simulink model "ex9busSG_sim"  (R2014b)
settings: Solver=ode45  SolverMode=SingleTasking  StartTime=0.0  StopTime=6  MaxStep=0.006  RelTol=1e-05
values from neighbouring files (symbols this model uses):
  Ar = full(Ar)    [ex9busSG.m]
  baseA = baseVA/baseV    [ex14busSGandPV.m]    (also in ex9busSG.m; exDroopA.m = baseVA./baseV; exDroopB.m = baseVA./baseV; exLargeSysStability.m = baseVA./baseV)
  baseV = 1e3*mpcA.bus(1,BASE_KV)    [ex14busSGandPV.m]    (also in ex9busSG_data.mat = 345000; exDroopA.m = 1e3*mpc.bus(:,BASE_KV); exDroopB.m = 1e3*mpc.bus(:,BASE_KV); exLargeSysStability.m = 1e3*mpc.bus(:,BASE_KV))
  baseVA = mpcA.baseMVA * 1e6    [ex14busSGandPV.m]    (also in ex9busSG.m = mpc.baseMVA*1e6; exDroopA.m = mpc.baseMVA * 1e6; exDroopB.m = mpc.baseMVA * 1e6; exLargeSysStability.m = mpc.baseMVA * 1e6)
  Br = full(Br)    [ex9busSG.m]
  Cr = full(Cr)    [ex9busSG.m]
  delta_init = mpc.bus(Genbus,VA)*pi/180    [ex9busSG.m]
  Dr = full(Dr)    [ex9busSG.m]
  Genbus = Genbus(2:end)    [ex9busSG.m]
  Kd = KD_GAIN_CNST*J*ws    [ex14busSGandPV.m]    (also in ex2busStability.m = 24000; ex7busLongLine.m; ex9busSG.m; exDroopA.m)
  lamda = (2^0.5) * Vgmag/ws    (= 45.916132124)    [ex2busStability.m]    (also in ex9busSG.m = (2^0.5) * Vn_gens/ws)
  MM = length(ssbus)    [ex9busSG.m]    (also in exLargeSysStability.m)
  poles_2Jws = poles./(2*J*ws)    [ex14busSGandPV.m]    (also in ex2busStability.m = poles./(2*ws*J); ex7busLongLine.m; ex9busSG.m = poles./(2*ws*J); exDroopA.m)
  ppm_default = (3*Pn_gens)    [ex9busSG.m]
  ppm_step_size_W = ppm_rel_step*Pmax_gens(which_generator_to_step)    [ex9busSG.m]
  ppm_step_time = 2    [ex9busSG.m]
  ref_vd_MKS = (2^0.5)*real(VV1ph)    [ex9busSG.m]
  ref_vq_MKS = (2^0.5)*imag(VV1ph)    [ex9busSG.m]
  ws = 2*pi*50    (= 314.159265359)    [ex14busSGandPV.m]    (also in ex2busStability.m; ex3busPV.m; ex7busLongLine.m; ex9busSG.m)
libraries: simulink x2
settings Model: Creator=COPEC  LastModifiedBy=Juri
settings OptimizationCC: BlockReduction=off  BooleanDataType=off
settings DebuggingCC: SaveWithParameterizedLinksMsg=none  UnderspecifiedInitializationDetection=Classic  MergeDetectMultiDrivingBlocksExec=none  SignalResolutionControl=TryResolveAllWithWarning  SolverPrmCheckMsg=none  FrameProcessingCompatibilityMsg=error
settings HardwareCC: TargetUnknown=on

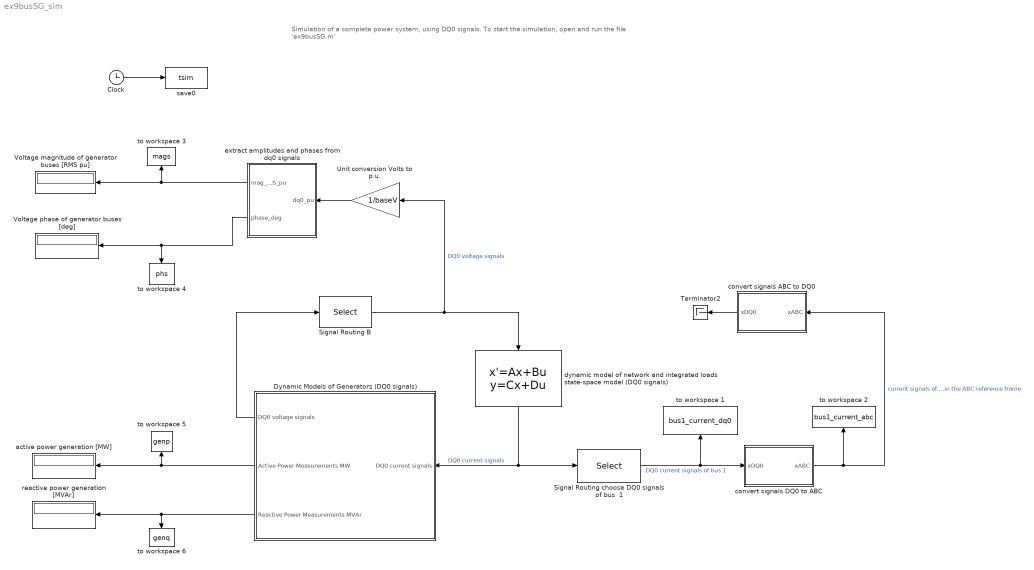
== system ex9busSG_sim ==
  note: Simulation of a complete power system, using DQ0 signals.
      |
      | To start the simulation, open and run the file
      | 'ex9busSG.m'
  Clock : Clock
  Dynamic Models of Generators (DQ0 signals) : Subsystem
  "Signal Routing choose DQ0 signals of bus  1 " : Selector  InputPortWidth=3*MM  IndexOptions=Index vector (dialog)  Indices=Bus_to_Ref  OutputSizes=1
  Signal Routing B : Selector  InputPortWidth=3*MM  IndexOptions=Index vector (dialog)  Indices=Units_to_Net  OutputSizes=1
  Terminator2 : Terminator
  Unit conversion Volts to p.u. : Gain  Gain=1/baseV
  Voltage magnitude of generator buses [RMS pu] : Display
  Voltage phase of generator buses [deg] : Display
  active power generation [MW] : Display
  convert signals ABC to DQ0 : Subsystem
  convert signals DQ0 to ABC : Subsystem
  dynamic model of network and integrated loads state-space model (DQ0 signals) : StateSpace  A=Ar  B=Br  C=Cr  D=Dr  X0=0
  extract amplitudes and phases from dq0 signals : Subsystem
  reactive power generation [MVAr] : Display
  save0 : ToWorkspace  VariableName=tsim  SampleTime=-1
  to workspace 1 : ToWorkspace  VariableName=bus1_current_dq0  SampleTime=-1
  to workspace 2 : ToWorkspace  VariableName=bus1_current_abc  SampleTime=-1
  to workspace 3 : ToWorkspace  VariableName=mags  SampleTime=-1
  to workspace 4 : ToWorkspace  VariableName=phs  SampleTime=-1
  to workspace 5 : ToWorkspace  VariableName=genp  SampleTime=-1
  to workspace 6 : ToWorkspace  VariableName=genq  SampleTime=-1
  wires:
  Clock/1 -> save0/1
  extract amplitudes and phases from dq0 signals/2(phase_deg) -> to workspace 4/1, Voltage phase of generator buses [deg]/1
  extract amplitudes and phases from dq0 signals/1(mag_RMS_pu) -> to workspace 3/1, Voltage magnitude of generator buses [RMS pu]/1
  Unit conversion Volts to p.u./1 -> extract amplitudes and phases from dq0 signals/1(dq0_pu)
  dynamic model of network and integrated loads state-space model (DQ0 signals)/1 -> "Signal Routing choose DQ0 signals of bus  1 "/1, Dynamic Models of Generators (DQ0 signals)/1(DQ0 current signals)  "DQ0 current signals"
  Signal Routing B/1 -> Unit conversion Volts to p.u./1, dynamic model of network and integrated loads state-space model (DQ0 signals)/1  "DQ0 voltage signals"
  "Signal Routing choose DQ0 signals of bus  1 "/1 -> convert signals DQ0 to ABC/1(xDQ0), to workspace 1/1  "DQ0 current signals of bus 1"
  convert signals DQ0 to ABC/1(xABC) -> convert signals ABC to DQ0/1(xABC), to workspace 2/1  "current signals of bus 1 in the ABC reference frame"
  convert signals ABC to DQ0/1(xDQ0) -> Terminator2/1
  Dynamic Models of Generators (DQ0 signals)/3(Reactive Power Measurements MVAr) -> reactive power generation [MVAr]/1, to workspace 6/1
  Dynamic Models of Generators (DQ0 signals)/2(Active Power Measurements MW) -> active power generation [MW]/1, to workspace 5/1
  Dynamic Models of Generators (DQ0 signals)/1(DQ0 voltage signals) -> Signal Routing B/1

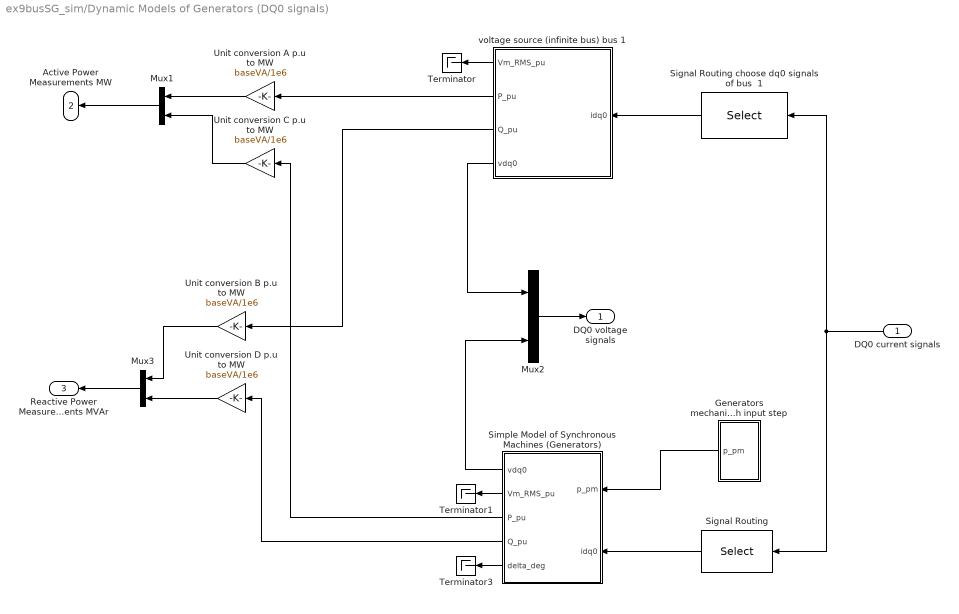
== system ex9busSG_sim/Dynamic Models of Generators (DQ0 signals) ==
  DQ0 current signals : Inport
  Generators mechanical powers with input step : Subsystem
  Mux1 : Mux  Inputs=2
  Mux2 : Mux  Inputs=2
  Mux3 : Mux  Inputs=2
  Signal Routing : Selector  InputPortWidth=3*MM  IndexOptions=Index vector (dialog)  Indices=Bus_to_Gen  OutputSizes=1
  "Signal Routing choose dq0 signals of bus  1 " : Selector  InputPortWidth=3*MM  IndexOptions=Index vector (dialog)  Indices=Bus_to_Ref  OutputSizes=1
  Simple Model of Synchronous Machines (Generators) : Subsystem
  Terminator : Terminator
  Terminator1 : Terminator
  Terminator3 : Terminator
  Unit conversion A p.u to MW : Gain  Gain=baseVA/1e6
  Unit conversion B p.u to MW : Gain  Gain=baseVA/1e6
  Unit conversion C p.u to MW : Gain  Gain=baseVA/1e6
  Unit conversion D p.u to MW : Gain  Gain=baseVA/1e6
  voltage source (infinite bus) bus 1 : Subsystem
  DQ0 voltage signals : Outport
  Active Power Measurements MW : Outport  Port=2
  Reactive Power Measurements MVAr : Outport  Port=3
  wires:
  voltage source (infinite bus) bus 1/2(P_pu) -> Unit conversion A p.u to MW/1
  Simple Model of Synchronous Machines (Generators)/4(Q_pu) -> Unit conversion D p.u to MW/1
  voltage source (infinite bus) bus 1/1(Vm_RMS_pu) -> Terminator/1
  Mux2/1 -> DQ0 voltage signals/1
  Signal Routing/1 -> Simple Model of Synchronous Machines (Generators)/2(idq0)
  voltage source (infinite bus) bus 1/4(vdq0) -> Mux2/1
  Simple Model of Synchronous Machines (Generators)/1(vdq0) -> Mux2/2
  "Signal Routing choose dq0 signals of bus  1 "/1 -> voltage source (infinite bus) bus 1/1(idq0)
  Unit conversion A p.u to MW/1 -> Mux1/1
  Unit conversion B p.u to MW/1 -> Mux3/1
  Simple Model of Synchronous Machines (Generators)/5(delta_deg) -> Terminator3/1
  Simple Model of Synchronous Machines (Generators)/2(Vm_RMS_pu) -> Terminator1/1
  Mux3/1 -> Reactive Power Measurements MVAr/1
  Unit conversion D p.u to MW/1 -> Mux3/2
  Unit conversion C p.u to MW/1 -> Mux1/2
  Mux1/1 -> Active Power Measurements MW/1
  Simple Model of Synchronous Machines (Generators)/3(P_pu) -> Unit conversion C p.u to MW/1
  DQ0 current signals/1 -> "Signal Routing choose dq0 signals of bus  1 "/1, Signal Routing/1
  voltage source (infinite bus) bus 1/3(Q_pu) -> Unit conversion B p.u to MW/1
  Generators mechanical powers with input step/1(p_pm) -> Simple Model of Synchronous Machines (Generators)/1(p_pm)

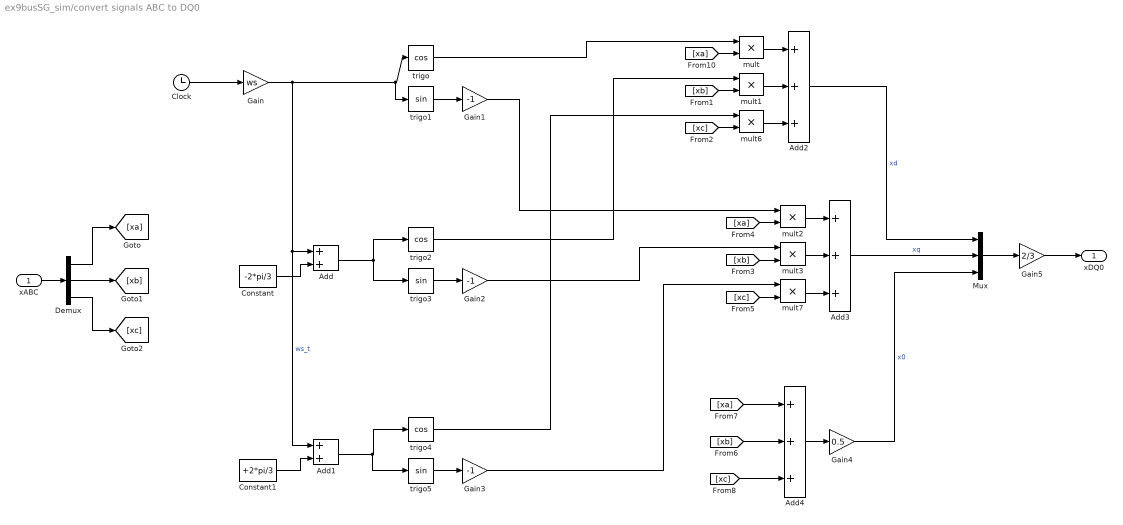
== system ex9busSG_sim/convert signals ABC to DQ0 ==
  xABC : Inport
  Add : Sum
  Add1 : Sum
  Add2 : Sum  Inputs=+++
  Add3 : Sum  Inputs=+++
  Add4 : Sum  Inputs=+++
  Clock : Clock
  Constant : Constant  Value=-2*pi/3
  Constant1 : Constant  Value=+2*pi/3
  Demux : Demux  Outputs=3
  Gain : Gain  Gain=ws
  Gain1 : Gain  Gain=-1
  Gain2 : Gain  Gain=-1
  Gain3 : Gain  Gain=-1
  Gain4 : Gain  Gain=0.5
  Gain5 : Gain  Gain=2/3
  Mux : Mux  Inputs=3
  mult{,1..3,6..7} (6 alike) : Product  Inputs=**
  trigo : Trigonometry  Operator=cos
  trigo1 : Trigonometry
  trigo2 : Trigonometry  Operator=cos
  trigo3 : Trigonometry
  trigo4 : Trigonometry  Operator=cos
  trigo5 : Trigonometry
  xDQ0 : Outport
  wires:
  Clock/1 -> Gain/1
  Gain/1 -> trigo1/1, trigo/1, Add1/1, Add/1  "ws_t"
  Constant/1 -> Add/2
  Constant1/1 -> Add1/2
  trigo1/1 -> Gain1/1
  trigo3/1 -> Gain2/1
  Add/1 -> trigo2/1, trigo3/1
  trigo5/1 -> Gain3/1
  Add1/1 -> trigo5/1, trigo4/1
  xABC/1 -> Demux/1
  Demux/1 -> [xa]
  Demux/2 -> [xb]
  Demux/3 -> [xc]
  mult/1 -> Add2/1
  mult1/1 -> Add2/2
  [xa] -> mult/2
  [xb] -> mult1/2
  mult2/1 -> Add3/1
  mult3/1 -> Add3/2
  Add2/1 -> Mux/1  "xd"
  Add3/1 -> Mux/2  "xq"
  Gain4/1 -> Mux/3  "x0"
  trigo/1 -> mult/1
  trigo2/1 -> mult1/1
  [xc] -> mult6/2
  mult6/1 -> Add2/3
  trigo4/1 -> mult6/1
  [xa] -> mult2/2
  [xb] -> mult3/2
  [xc] -> mult7/2
  mult7/1 -> Add3/3
  Add4/1 -> Gain4/1
  [xa] -> Add4/1
  [xb] -> Add4/2
  [xc] -> Add4/3
  Gain1/1 -> mult2/1
  Gain2/1 -> mult3/1
  Gain3/1 -> mult7/1
  Mux/1 -> Gain5/1
  Gain5/1 -> xDQ0/1

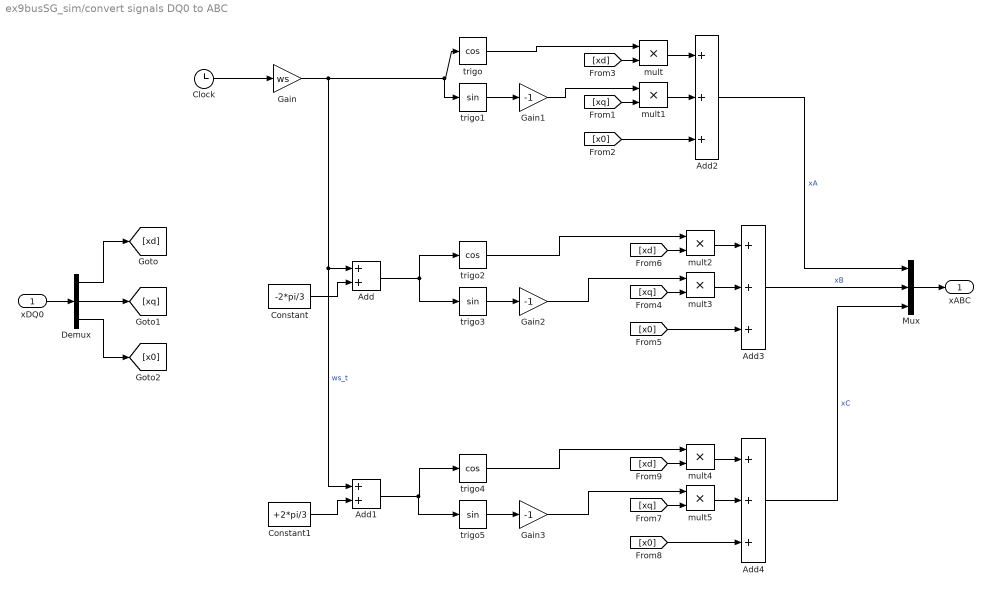
== system ex9busSG_sim/convert signals DQ0 to ABC ==
  xDQ0 : Inport
  Add : Sum
  Add1 : Sum
  Add2 : Sum  Inputs=+++
  Add3 : Sum  Inputs=+++
  Add4 : Sum  Inputs=+++
  Clock : Clock
  Constant : Constant  Value=-2*pi/3
  Constant1 : Constant  Value=+2*pi/3
  Demux : Demux  Outputs=3
  Gain : Gain  Gain=ws
  Gain1 : Gain  Gain=-1
  Gain2 : Gain  Gain=-1
  Gain3 : Gain  Gain=-1
  Mux : Mux  Inputs=3
  mult{,1..5} (6 alike) : Product  Inputs=**
  trigo : Trigonometry  Operator=cos
  trigo1 : Trigonometry
  trigo2 : Trigonometry  Operator=cos
  trigo3 : Trigonometry
  trigo4 : Trigonometry  Operator=cos
  trigo5 : Trigonometry
  xABC : Outport
  wires:
  Clock/1 -> Gain/1
  Gain/1 -> trigo1/1, trigo/1, Add1/1, Add/1  "ws_t"
  Constant/1 -> Add/2
  Constant1/1 -> Add1/2
  trigo1/1 -> Gain1/1
  trigo3/1 -> Gain2/1
  Add/1 -> trigo2/1, trigo3/1
  trigo5/1 -> Gain3/1
  Add1/1 -> trigo5/1, trigo4/1
  xDQ0/1 -> Demux/1
  Demux/1 -> [xd]
  Demux/2 -> [xq]
  Demux/3 -> [x0]
  Mux/1 -> xABC/1
  mult/1 -> Add2/1
  mult1/1 -> Add2/2
  [xd] -> mult/2
  [xq] -> mult1/2
  [x0] -> Add2/3
  mult2/1 -> Add3/1
  mult3/1 -> Add3/2
  [xd] -> mult2/2
  [xq] -> mult3/2
  [x0] -> Add3/3
  mult4/1 -> Add4/1
  mult5/1 -> Add4/2
  [xd] -> mult4/2
  [xq] -> mult5/2
  [x0] -> Add4/3
  trigo/1 -> mult/1
  Gain1/1 -> mult1/1
  trigo2/1 -> mult2/1
  Gain2/1 -> mult3/1
  trigo4/1 -> mult4/1
  Gain3/1 -> mult5/1
  Add2/1 -> Mux/1  "xA"
  Add3/1 -> Mux/2  "xB"
  Add4/1 -> Mux/3  "xC"

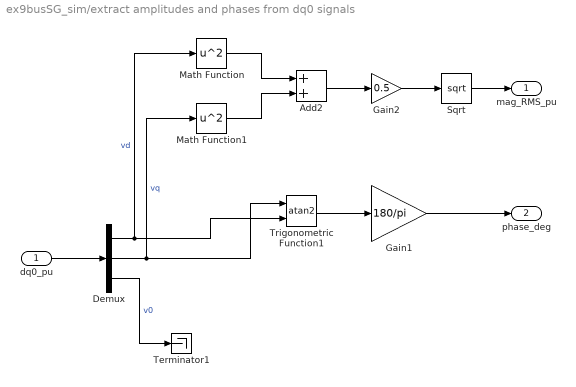
== system ex9busSG_sim/extract amplitudes and phases from dq0 signals ==
  dq0_pu : Inport
  Add2 : Sum
  Demux : Demux  Outputs=3
  Gain1 : Gain  Gain=180/pi
  Gain2 : Gain  Gain=0.5
  Math Function : Math  Operator=square  SaturateOnIntegerOverflow=on
  Math Function1 : Math  Operator=square  SaturateOnIntegerOverflow=on
  Sqrt : Sqrt  SaturateOnIntegerOverflow=on
  Terminator1 : Terminator
  Trigonometric Function1 : Trigonometry  Operator=atan2
  mag_RMS_pu : Outport
  phase_deg : Outport  Port=2
  wires:
  dq0_pu/1 -> Demux/1
  Demux/1 -> Trigonometric Function1/2, Math Function/1  "vd"
  Demux/2 -> Trigonometric Function1/1, Math Function1/1  "vq"
  Demux/3 -> Terminator1/1  "v0"
  Sqrt/1 -> mag_RMS_pu/1
  Math Function/1 -> Add2/1
  Math Function1/1 -> Add2/2
  Add2/1 -> Gain2/1
  Gain2/1 -> Sqrt/1
  Trigonometric Function1/1 -> Gain1/1
  Gain1/1 -> phase_deg/1

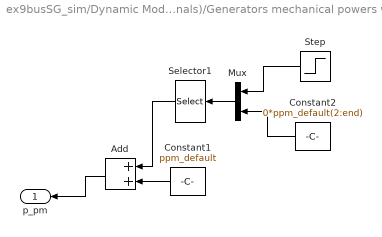
== system ex9busSG_sim/Dynamic Models of Generators (DQ0 signals)/Generators mechanical powers with input step ==
  Add : Sum
  Constant1 : Constant  Value=ppm_default
  Constant2 : Constant  Value=0*ppm_default(2:end)
  Mux : Mux  Inputs=2
  Selector1 : Selector  InputPortWidth=length(ppm_default)  IndexOptions=Index vector (dialog)  Indices=step_index_vector  OutputSizes=1
  Step : Step  Time=ppm_step_time  After=ppm_step_size_W  SampleTime=0
  p_pm : Outport
  wires:
  Constant1/1 -> Add/2
  Selector1/1 -> Add/1
  Constant2/1 -> Mux/2
  Mux/1 -> Selector1/1
  Step/1 -> Mux/1
  Add/1 -> p_pm/1

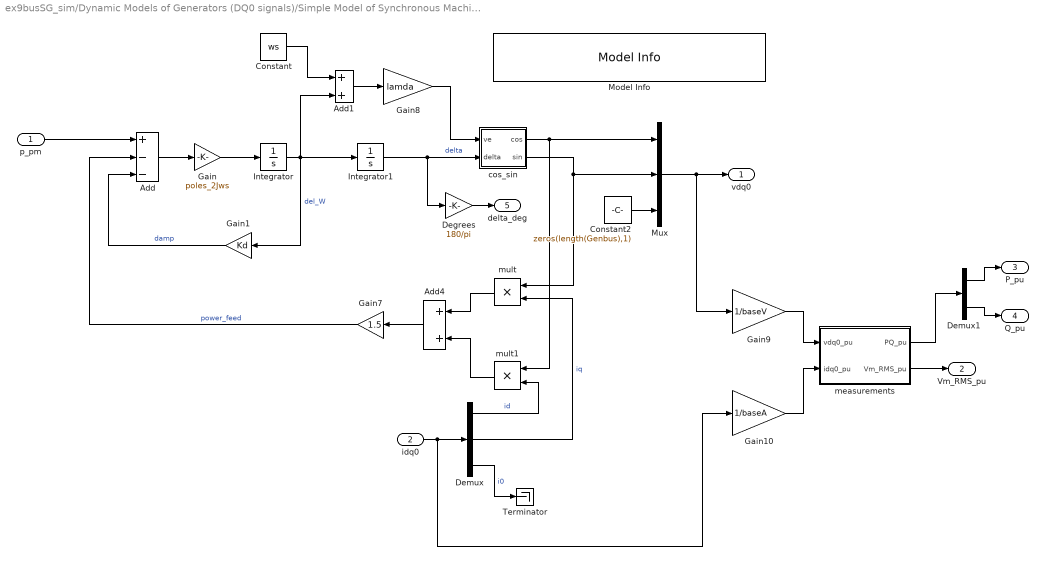
== system ex9busSG_sim/Dynamic Models of Generators (DQ0 signals)/Simple Model of Synchronous Machines (Generators) ==
  p_pm : Inport
  idq0 : Inport  Port=2
  Add : Sum  Inputs=+--
  Add1 : Sum
  Add4 : Sum
  Constant : Constant  Value=ws
  Constant2 : Constant  Value=zeros(length(Genbus),1)
  Degrees : Gain  Gain=180/pi
  Demux : Demux  Outputs=3
  Demux1 : Demux  Outputs=2
  Gain : Gain  Gain=poles_2Jws
  Gain1 : Gain  Gain=Kd
  Gain10 : Gain  Gain=1/baseA
  Gain7 : Gain  Gain=1.5
  Gain8 : Gain  Gain=lamda
  Gain9 : Gain  Gain=1/baseV
  Integrator : Integrator
  Integrator1 : Integrator  InitialCondition=delta_init
  Model Info : simulink/Model-Wide Utilities/Model Info  Frame=on  DisplayStringWithTags=Model Info  HorizontalTextAlignment=Center  LeftAlignmentValue=0.5  SourceBlockDiagram=ex9busSG_sim  TagMaxNumber=20
  Mux : Mux  Inputs=3
  Terminator : Terminator
  cos_sin : Subsystem
  measurements : Subsystem
  mult : Product  Inputs=**
  mult1 : Product  Inputs=**
  vdq0 : Outport
  Vm_RMS_pu : Outport  Port=2
  P_pu : Outport  Port=3
  Q_pu : Outport  Port=4
  delta_deg : Outport  Port=5
  wires:
  p_pm/1 -> Add/1
  Add/1 -> Gain/1
  Gain/1 -> Integrator/1
  Integrator/1 -> Add1/2, Gain1/1, Integrator1/1  "del_W"
  Integrator1/1 -> cos_sin/2(delta), Degrees/1  "delta"
  Gain1/1 -> Add/3  "damp"
  Demux/3 -> Terminator/1  "i0"
  cos_sin/1(cos) -> mult1/1, Mux/1
  cos_sin/2(sin) -> mult/1, Mux/2
  mult/1 -> Add4/1
  mult1/1 -> Add4/2
  Add4/1 -> Gain7/1
  Gain7/1 -> Add/2  "power_feed"
  idq0/1 -> Gain10/1, Demux/1
  Mux/1 -> Gain9/1, vdq0/1
  Add1/1 -> Gain8/1
  Degrees/1 -> delta_deg/1
  Gain8/1 -> cos_sin/1(ve)
  Constant/1 -> Add1/1
  measurements/2(Vm_RMS_pu) -> Vm_RMS_pu/1
  Gain9/1 -> measurements/1(vdq0_pu)
  Gain10/1 -> measurements/2(idq0_pu)
  Constant2/1 -> Mux/3
  Demux/1 -> mult1/2  "id"
  Demux/2 -> mult/2  "iq"
  measurements/1(PQ_pu) -> Demux1/1
  Demux1/1 -> P_pu/1
  Demux1/2 -> Q_pu/1

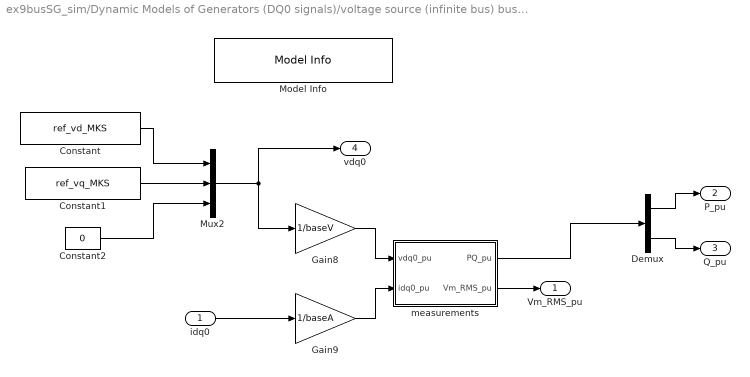
== system ex9busSG_sim/Dynamic Models of Generators (DQ0 signals)/voltage source (infinite bus) bus 1 ==
  idq0 : Inport
  Constant : Constant  Value=ref_vd_MKS
  Constant1 : Constant  Value=ref_vq_MKS
  Constant2 : Constant  Value=0
  Demux : Demux  Outputs=2
  Gain8 : Gain  Gain=1/baseV
  Gain9 : Gain  Gain=1/baseA
  Model Info : simulink/Model-Wide Utilities/Model Info  Frame=on  DisplayStringWithTags=Model Info  HorizontalTextAlignment=Center  LeftAlignmentValue=0.5  SourceBlockDiagram=ex9busSG_sim  TagMaxNumber=20
  Mux2 : Mux  Inputs=3
  measurements : Subsystem
  Vm_RMS_pu : Outport
  P_pu : Outport  Port=2
  Q_pu : Outport  Port=3
  vdq0 : Outport  Port=4
  wires:
  Constant/1 -> Mux2/1
  Constant1/1 -> Mux2/2
  Constant2/1 -> Mux2/3
  Mux2/1 -> Gain8/1, vdq0/1
  idq0/1 -> Gain9/1
  measurements/1(PQ_pu) -> Demux/1
  measurements/2(Vm_RMS_pu) -> Vm_RMS_pu/1
  Gain8/1 -> measurements/1(vdq0_pu)
  Gain9/1 -> measurements/2(idq0_pu)
  Demux/1 -> P_pu/1
  Demux/2 -> Q_pu/1

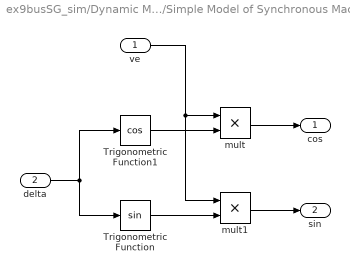
== system ex9busSG_sim/Dynamic Models of Generators (DQ0 signals)/Simple Model of Synchronous Machines (Generators)/cos_sin ==
  ve : Inport
  delta : Inport  Port=2
  Trigonometric Function : Trigonometry
  Trigonometric Function1 : Trigonometry  Operator=cos
  mult : Product  Inputs=**
  mult1 : Product  Inputs=**
  cos : Outport
  sin : Outport  Port=2
  wires:
  delta/1 -> Trigonometric Function/1, Trigonometric Function1/1
  Trigonometric Function1/1 -> mult/2
  ve/1 -> mult1/1, mult/1
  Trigonometric Function/1 -> mult1/2
  mult/1 -> cos/1
  mult1/1 -> sin/1

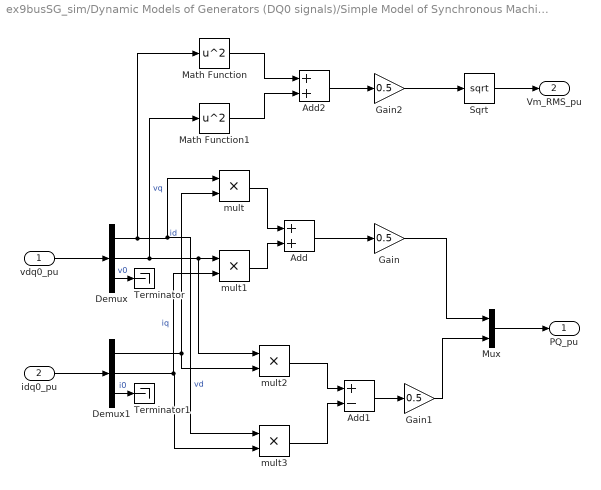
== system ex9busSG_sim/Dynamic Models of Generators (DQ0 signals)/Simple Model of Synchronous Machines (Generators)/measurements ==
  vdq0_pu : Inport
  idq0_pu : Inport  Port=2
  Add : Sum
  Add1 : Sum  Inputs=+-
  Add2 : Sum
  Demux : Demux  Outputs=3
  Demux1 : Demux  Outputs=3
  Gain : Gain  Gain=0.5
  Gain1 : Gain  Gain=0.5
  Gain2 : Gain  Gain=0.5
  Math Function : Math  Operator=square  SaturateOnIntegerOverflow=on
  Math Function1 : Math  Operator=square  SaturateOnIntegerOverflow=on
  Mux : Mux  Inputs=2
  Sqrt : Sqrt  SaturateOnIntegerOverflow=on
  Terminator : Terminator
  Terminator1 : Terminator
  mult{,1..3} (4 alike) : Product  Inputs=**
  PQ_pu : Outport
  Vm_RMS_pu : Outport  Port=2
  wires:
  Mux/1 -> PQ_pu/1
  idq0_pu/1 -> Demux1/1
  vdq0_pu/1 -> Demux/1
  Demux/1 -> Math Function/1, mult3/1, mult/1  "vd"
  Demux/2 -> Math Function1/1, mult2/1, mult1/1  "vq"
  Demux1/1 -> mult/2, mult2/2  "id"
  Demux1/2 -> mult3/2, mult1/2  "iq"
  Demux/3 -> Terminator/1  "v0"
  Demux1/3 -> Terminator1/1  "i0"
  mult/1 -> Add/1
  mult1/1 -> Add/2
  Add/1 -> Gain/1
  Gain/1 -> Mux/1
  mult2/1 -> Add1/1
  mult3/1 -> Add1/2
  Add1/1 -> Gain1/1
  Gain1/1 -> Mux/2
  Sqrt/1 -> Vm_RMS_pu/1
  Math Function/1 -> Add2/1
  Math Function1/1 -> Add2/2
  Add2/1 -> Gain2/1
  Gain2/1 -> Sqrt/1

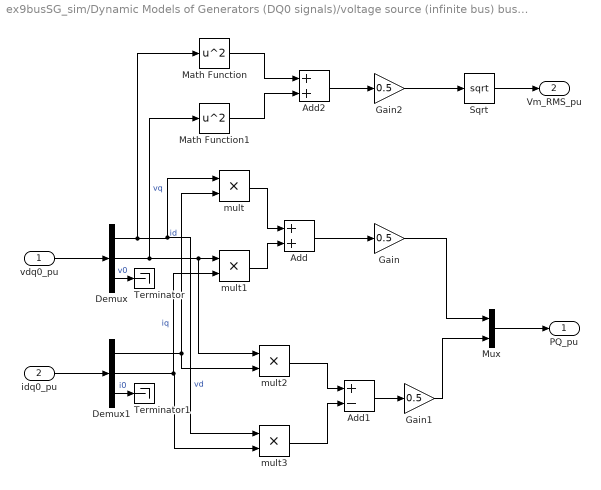
== system ex9busSG_sim/Dynamic Models of Generators (DQ0 signals)/voltage source (infinite bus) bus 1/measurements ==
  vdq0_pu : Inport
  idq0_pu : Inport  Port=2
  Add : Sum
  Add1 : Sum  Inputs=+-
  Add2 : Sum
  Demux : Demux  Outputs=3
  Demux1 : Demux  Outputs=3
  Gain : Gain  Gain=0.5
  Gain1 : Gain  Gain=0.5
  Gain2 : Gain  Gain=0.5
  Math Function : Math  Operator=square  SaturateOnIntegerOverflow=on
  Math Function1 : Math  Operator=square  SaturateOnIntegerOverflow=on
  Mux : Mux  Inputs=2
  Sqrt : Sqrt  SaturateOnIntegerOverflow=on
  Terminator : Terminator
  Terminator1 : Terminator
  mult{,1..3} (4 alike) : Product  Inputs=**
  PQ_pu : Outport
  Vm_RMS_pu : Outport  Port=2
  wires:
  Mux/1 -> PQ_pu/1
  idq0_pu/1 -> Demux1/1
  vdq0_pu/1 -> Demux/1
  Demux/1 -> Math Function/1, mult3/1, mult/1  "vd"
  Demux/2 -> Math Function1/1, mult2/1, mult1/1  "vq"
  Demux1/1 -> mult/2, mult2/2  "id"
  Demux1/2 -> mult3/2, mult1/2  "iq"
  Demux/3 -> Terminator/1  "v0"
  Demux1/3 -> Terminator1/1  "i0"
  mult/1 -> Add/1
  mult1/1 -> Add/2
  Add/1 -> Gain/1
  Gain/1 -> Mux/1
  mult2/1 -> Add1/1
  mult3/1 -> Add1/2
  Add1/1 -> Gain1/1
  Gain1/1 -> Mux/2
  Sqrt/1 -> Vm_RMS_pu/1
  Math Function/1 -> Add2/1
  Math Function1/1 -> Add2/2
  Add2/1 -> Gain2/1
  Gain2/1 -> Sqrt/1
